simulink subsystem "RMS"  (R2020b)
settings: Solver=VariableStepAuto  StartTime=0.0  StopTime=10.0  RelTol=1e-3
settings Model: Creator=marco  LastModifiedBy=marco

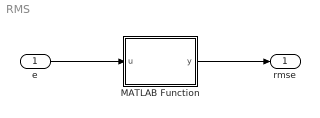
== system RMS ==
  e : Inport
  MATLAB Function : MATLAB Function  TreatAsAtomicUnit=on
  rmse : Outport
  wires:
  e/1 -> MATLAB Function/1(u)
  MATLAB Function/1(y) -> rmse/1

== matlab function RMS/MATLAB Function ==
  data: u input; y output
function y = fcn(u)

y = norm(u)/sqrt(numel(u)/3);
